simulink model "Circuit4"  (R2022a)
settings: Solver=VariableStepAuto  StartTime=0.0  StopTime=10.0  RelTol=1e-3
libraries: fl_lib x7, nesl_utility x2
settings Model: Creator=bdawg  LastModifiedBy=bdawg

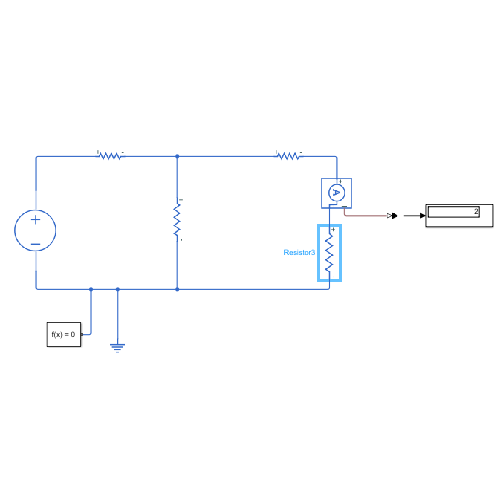
[thumbnail: Simulink's stored preview of the top-level diagram]
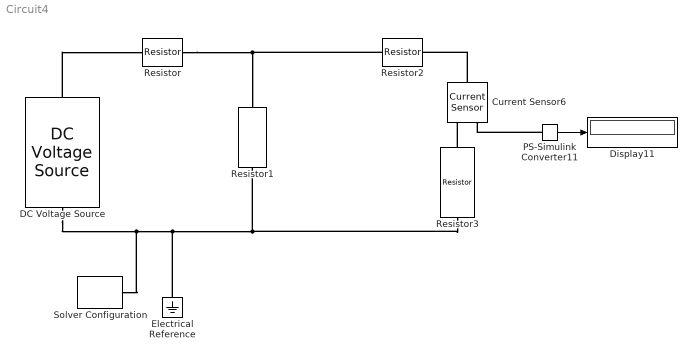
== system Circuit4 ==
  Current Sensor6 : fl_lib/Electrical/Electrical Sensors/Current Sensor
      settings: SourceProductBaseCode=PW,SS,VE
  DC Voltage Source : fl_lib/Electrical/Electrical Sources/DC Voltage Source  v0=60 V
      settings: SourceProductBaseCode=PW,SS,VE
  Display11 : Display
  Electrical Reference : fl_lib/Electrical/Electrical Elements/Electrical Reference
      settings: SourceProductBaseCode=PW,SS,VE
  PS-Simulink Converter11 : nesl_utility/PS-Simulink Converter  PhysicalDomain=network_engine_domain  SubClassName=ps_output  LeftPortType=input  RightPortType=output  PseudoPeriodic=off  Frequencies=[]  VectorFormat=inherit  Unit=inherit  AffineConversion=off
      settings: SourceProductBaseCode=SS,PW,VE
  Resistor : fl_lib/Electrical/Electrical Elements/Resistor  R=10 Ohm  i_specify=off  i_priority=None  i=0 A  i_nominal_specify=off  i_nominal_unit=A  i_nominal_value=1  v_specify=off  v_priority=None  v=0 V  v_nominal_specify=off  v_nominal_unit=V  v_nominal_value=1
      settings: SourceProductBaseCode=PW,SS,VE
  Resistor1 : fl_lib/Electrical/Electrical Elements/Resistor  R=40 Ohm  i_specify=off  i_priority=None  i=0 A  i_nominal_specify=off  i_nominal_unit=A  i_nominal_value=1  v_specify=off  v_priority=None  v=0 V  v_nominal_specify=off  v_nominal_unit=V  v_nominal_value=1
      settings: SourceProductBaseCode=PW,SS,VE
  Resistor2 : fl_lib/Electrical/Electrical Elements/Resistor  R=8 Ohm  i_specify=off  i_priority=None  i=0 A  i_nominal_specify=off  i_nominal_unit=A  i_nominal_value=1  v_specify=off  v_priority=None  v=0 V  v_nominal_specify=off  v_nominal_unit=V  v_nominal_value=1
      settings: SourceProductBaseCode=PW,SS,VE
  Resistor3 : fl_lib/Electrical/Electrical Elements/Resistor  R=8 Ohm  i_specify=off  i_priority=None  i=0 A  i_nominal_specify=off  i_nominal_unit=A  i_nominal_value=1  v_specify=off  v_priority=None  v=0 V  v_nominal_specify=off  v_nominal_unit=V  v_nominal_value=1
      settings: SourceProductBaseCode=PW,SS,VE
  Solver Configuration : nesl_utility/Solver Configuration  PhysicalDomain=network_engine_domain  SubClassName=solver  LeftPortType=input  RightPortType=generic  Tones=[]  Harmonics=[]  SimulateNoise=off  Profile=off  UseLocalSampling=off  EnableSwitchedLinearOptims=on  FrequencyDomain=off  UseCCode=off  RelTol=0.001  AbsTol=0.001  MinStep=1e-09  ToWorkspace=off  RevertToSquareIcSolve=off  NumHomotopyIterations=100  PhasorMode=off  PhasorModeNumHarmonics=1  IndexReductionMethod=DerivativeReplacement  DoDC=off  ResidualTolerance=1e-09  UseLocalSolver=off  LocalSolverChoice=NE_BACKWARD_EULER_ADVANCER  LocalSolverSampleTime=0.001  DoFixedCost=off  MaxNonlinIter=3  MaxModeIter=2  ComputeImpulses=off  ImpulseIterations=2  LinearAlgebra=auto  LinearAlgebraNumThread=0  EquationFormulation=NE_TIME_EF  DelaysMemoryBudget=1024  AutomaticFiltering=on  FilteringTimeConstant=0.001  PartitionStorageMethod=AS_NEEDED  PartitionMemoryBudget=1024  PartitionMethod=ROBUST
      settings: SourceProductBaseCode=SS,PW,VE
  wires:
  PS-Simulink Converter11/1 -> Display11/1
  connections:
  DC Voltage Source/LConn1 -- Resistor/LConn1
  Resistor/RConn1 -- Resistor1/LConn1 -- Resistor2/LConn1
  DC Voltage Source/RConn1 -- Solver Configuration/RConn1 -- Electrical Reference/LConn1 -- Resistor3/RConn1 -- Resistor1/RConn1
  Current Sensor6/LConn1 -- Resistor2/RConn1
  PS-Simulink Converter11/LConn1 -- Current Sensor6/RConn1
  Resistor3/LConn1 -- Current Sensor6/RConn2
